simulink model "ex5_model"  (R2013a)
settings: Solver=ode45  StartTime=0.0  StopTime=10.0  RelTol=1e-3
values from neighbouring files (symbols this model uses):
  c = 0.5    [ex5.m]
  C = 2    [ex5.m]
  k = 1    [ex5.m]    (also in ex6.m = 0.001)
  K = 49    [ex5.m]    (also in ex6.m = 1)
  m = 1    [ex5.m]    (also in ex6.m = 0.1)
  q1_0 = 0    [ex5.m]
  q1_dot_0 = 0    [ex5.m]
  q2_0 = 1    [ex5.m]
  q2_dot_0 = 0    [ex5.m]
settings Model: Creator=Brent  LastModifiedBy=Willdog

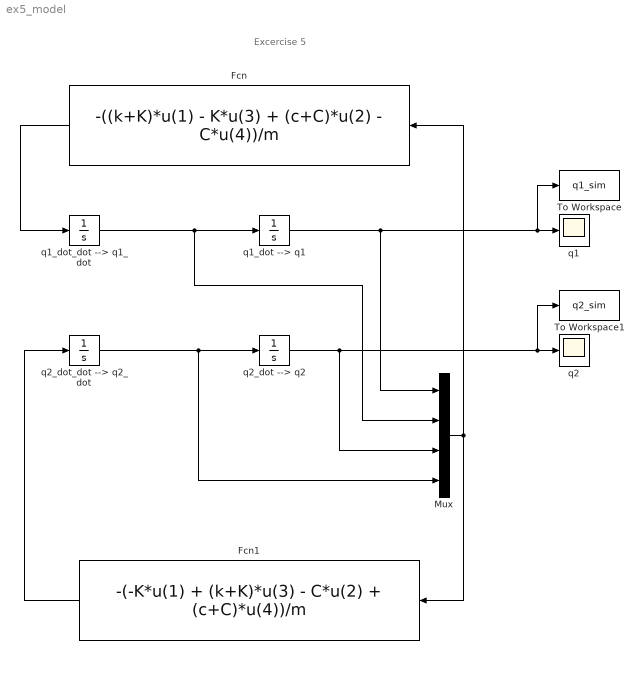
== system ex5_model ==
  note: Excercise 5
  Fcn : Fcn  Expr=-((k+K)*u(1) - K*u(3) + (c+C)*u(2) - C*u(4))/m
  Fcn1 : Fcn  Expr=-(-K*u(1) + (k+K)*u(3) - C*u(2) + (c+C)*u(4))/m
  Mux : Mux
  To Workspace : ToWorkspace  VariableName=q1_sim  SampleTime=-1  SaveFormat=Timeseries
  To Workspace1 : ToWorkspace  VariableName=q2_sim  SampleTime=-1  SaveFormat=Timeseries
  q1 : Scope
  q1_dot --> q1 : Integrator  InitialCondition=q1_0
  q1_dot_dot --> q1_dot : Integrator  InitialCondition=q1_dot_0
  q2 : Scope
  q2_dot --> q2 : Integrator  InitialCondition=q2_0
  q2_dot_dot --> q2_dot : Integrator  InitialCondition=q2_dot_0
  wires:
  q1_dot_dot --> q1_dot/1 -> q1_dot --> q1/1, Mux/2
  q2_dot_dot --> q2_dot/1 -> Mux/4, q2_dot --> q2/1
  q1_dot --> q1/1 -> Mux/1, To Workspace/1, q1/1
  q2_dot --> q2/1 -> To Workspace1/1, q2/1, Mux/3
  Mux/1 -> Fcn/1, Fcn1/1
  Fcn1/1 -> q2_dot_dot --> q2_dot/1
  Fcn/1 -> q1_dot_dot --> q1_dot/1
